simulink model "Cascade_1"  (R2021a)
settings: Solver=FixedStepDiscrete  StartTime=0.0  StopTime=10.0  FixedStep=0.2  RelTol=1e-3
settings Model: Creator=Utkarsh Anand  LastModifiedBy=Utkarsh Anand
settings DataIOCC: SaveOutput=off  SaveTime=off

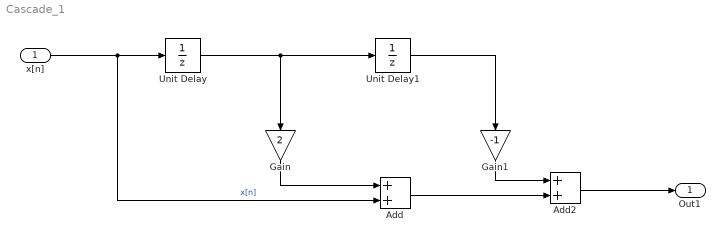
== system Cascade_1 ==
  x[n] : Inport  OutDataTypeStr=double  PortDimensions=1  SampleTime=[0.20000000000000001,0]
  Add : Sum
  Add2 : Sum
  Gain : Gain  Gain=2
  Gain1 : Gain  Gain=-1
  Unit Delay : UnitDelay  SampleTime=-1  HasFrameUpgradeWarning=on
  Unit Delay1 : UnitDelay  SampleTime=-1  HasFrameUpgradeWarning=on
  Out1 : Outport  OutDataTypeStr=double  PortDimensions=1  SampleTime=[0.20000000000000001,0]
  wires:
  Add/1 -> Add2/2
  Add2/1 -> Out1/1
  Unit Delay1/1 -> Gain1/1
  x[n]/1 -> Add/2, Unit Delay/1  "x[n]"
  Gain/1 -> Add/1
  Unit Delay/1 -> Gain/1, Unit Delay1/1
  Gain1/1 -> Add2/1
